simulink library "massSpringDamper_ul"  (R2022a)
settings: Solver=VariableStepAuto  StartTime=0.0  StopTime=10.0  RelTol=1e-3
settings Model: Creator=mcobb  LastModifiedBy=lhill8
settings SolverCC: AlgebraicLoopSolver=TrustRegion
settings DebuggingCC: UnconnectedInputMsg=warning  UnconnectedOutputMsg=warning  UnconnectedLineMsg=warning  SFMachineParentedDataDiag=warning  ArithmeticOperatorsInVariantConditions=warning
settings SFSimCC: CustomCodeUndefinedFunction=UseInterfaceOnly

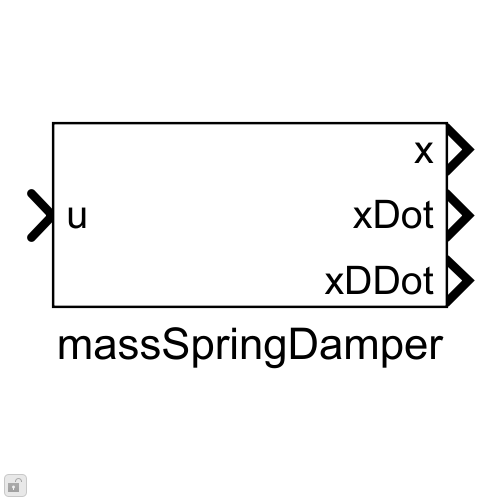
[thumbnail: Simulink's stored preview of the top-level diagram]
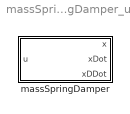
== system massSpringDamper_ul ==
  massSpringDamper : Subsystem  mask{m=1, b=1, k=1, x0=0, xDot0=0}
      mask prompts: m "Mass"; b "Damping Coefficient"; k "Spring Constant"; x0 "Initial Position"; xDot0 "Initial Velocity"
      mask DialogControl Container3 Prompt: Initial Conditions

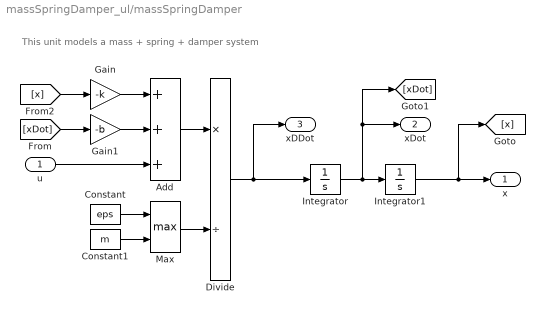
== system massSpringDamper_ul/massSpringDamper ==
  note: This unit models a mass + spring + damper system
  u : Inport
  Add : Sum  Inputs=+++
  Constant : Constant  Value=eps
  Constant1 : Constant  Value=m
  Divide : Product  Inputs=*/
  Gain : Gain  Gain=-k
  Gain1 : Gain  Gain=-b
  Integrator : Integrator  InitialCondition=xDot0
  Integrator1 : Integrator  InitialCondition=x0
  Max : MinMax  Function=max  Inputs=2
  x : Outport  VectorParamsAs1DForOutWhenUnconnected=off
  xDot : Outport  Port=2  VectorParamsAs1DForOutWhenUnconnected=off
  xDDot : Outport  Port=3  VectorParamsAs1DForOutWhenUnconnected=off
  wires:
  Max/1 -> Divide/2
  Constant/1 -> Max/1
  Divide/1 -> xDDot/1, Integrator/1
  Constant1/1 -> Max/2
  [x] -> Gain/1
  Gain/1 -> Add/1
  [xDot] -> Gain1/1
  Gain1/1 -> Add/2
  u/1 -> Add/3
  Add/1 -> Divide/1
  Integrator/1 -> xDot/1, [xDot], Integrator1/1
  Integrator1/1 -> x/1, [x]
